simulink model "myAdcDither"  (Simulink 7.3)
settings: Solver=FixedStepDiscrete  StartTime=0.0  StopTime=.1  RelTol=1e-3
values from neighbouring files (symbols this model uses):
  Ts = 1/(handles.clkFreq*1e6)*1e9    [myTimingAnalysis.m]
undefined symbols (not defined in the file or in its folder): overSamp
libraries: dspstat3 x3, commfilt2 x1, dspswit3 x1
settings Model: Creator=acarroll  LastModifiedBy=acarroll
settings DataIOCC: LimitDataPoints=off

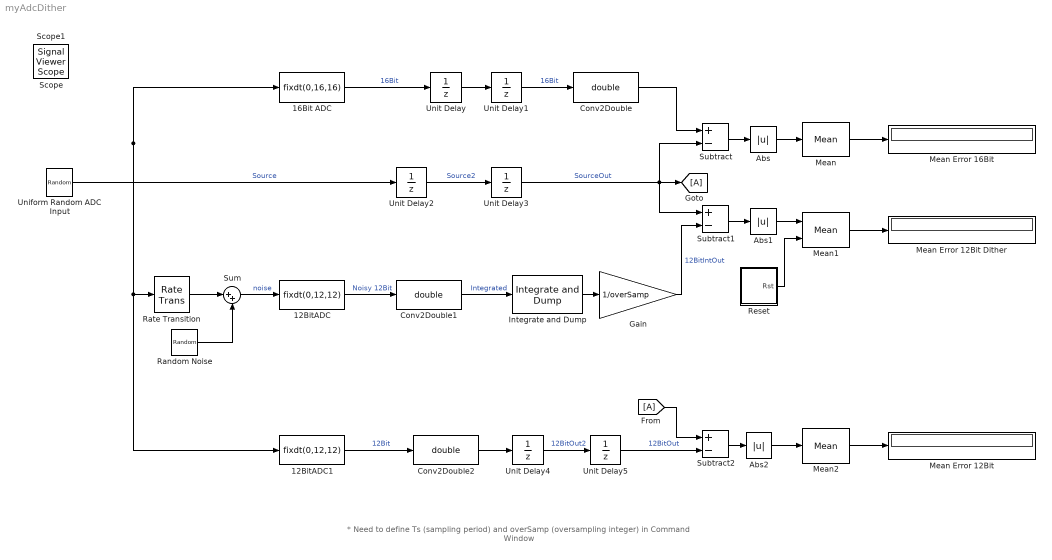
== system myAdcDither ==
  note: * Need to define Ts (sampling period) and overSamp (oversampling integer) in Command Window
  12BitADC : DataTypeConversion  OutDataTypeMode=Specify via dialog  OutDataType=fixdt(0,12,12)  OutDataTypeStr=fixdt(0,12,12)  RndMeth=Nearest  SampleTime=Ts/overSamp  SaturateOnIntegerOverflow=on
  12BitADC1 : DataTypeConversion  OutDataTypeMode=Specify via dialog  OutDataType=fixdt(0,12,12)  OutDataTypeStr=fixdt(0,12,12)  RndMeth=Nearest  SampleTime=Ts  SaturateOnIntegerOverflow=on
  16Bit ADC : DataTypeConversion  OutDataTypeMode=Specify via dialog  OutDataType=fixdt(0,16,16)  OutDataTypeStr=fixdt(0,16,16)  RndMeth=Nearest  SampleTime=Ts  SaturateOnIntegerOverflow=on
  Abs : Abs  OutDataType=fixdt(1, 16)  OutScaling=2^0
  Abs1 : Abs  OutDataType=fixdt(1, 16)  OutScaling=2^0
  Abs2 : Abs  OutDataType=fixdt(1, 16)  OutScaling=2^0
  Conv2Double : DataTypeConversion  OutDataTypeMode=double  OutDataType=fixdt(0,16,16)  OutDataTypeStr=double  SampleTime=Ts
  Conv2Double1 : DataTypeConversion  OutDataTypeMode=double  OutDataType=fixdt(0,16,16)  OutDataTypeStr=double
  Conv2Double2 : DataTypeConversion  OutDataTypeMode=double  OutDataType=fixdt(0,16,16)  OutDataTypeStr=double  SampleTime=Ts
  Gain : Gain  Gain=1/overSamp  ParameterDataType=fixdt(1, 16)  ParameterScaling=2^0  OutDataType=fixdt(1, 16)  OutScaling=2^0
  Integrate and Dump : commfilt2/Integrate and Dump  DialogController=commDDGCreate  DialogControllerArgs=DataTag0  obssamples=overSamp  offsetsamples=0  nodump=off  roundingMode=Convergent  overflowMode=on  outputMode=Binary point scaling  outputWordLength=64  outputFracLength=32
  Mean : dspstat3/Mean  DialogController=dspDDGCreate  DialogControllerArgs=DataTag1  run=on  reset_popup=None  directionMode=Each column  dimension=1  treatSBRowAsCol=on  roiEnable=off  roiType=Rectangles  roiPortion=Entire ROI  roiOutput=Individual statistics for each ROI  roiFlag=off  roundingMode=Floor  overflowMode=off
  Mean Error 12Bit : Display
  Mean Error 12Bit Dither : Display
  Mean Error 16Bit : Display
  Mean1 : dspstat3/Mean  DialogController=dspDDGCreate  DialogControllerArgs=DataTag2  run=on  reset_popup=Rising edge  directionMode=Each column  dimension=1  treatSBRowAsCol=on  roiEnable=off  roiType=Rectangles  roiPortion=Entire ROI  roiOutput=Individual statistics for each ROI  roiFlag=off  roundingMode=Floor  overflowMode=off
  Mean2 : dspstat3/Mean  DialogController=dspDDGCreate  DialogControllerArgs=DataTag3  run=on  reset_popup=None  directionMode=Each column  dimension=1  treatSBRowAsCol=on  roiEnable=off  roiType=Rectangles  roiPortion=Entire ROI  roiOutput=Individual statistics for each ROI  roiFlag=off  roundingMode=Floor  overflowMode=off
  Random Noise : RandomNumber  Variance=(.0002442/2)^2  Seed=5  SampleTime=Ts/overSamp
  Rate Transition : RateTransition
  Reset : Subsystem
  Subtract : Sum  Inputs=+-  OutDataType=fixdt(1, 16)  OutScaling=2^-10
  Subtract1 : Sum  Inputs=+-  OutDataType=fixdt(1, 16)  OutScaling=2^-10
  Subtract2 : Sum  Inputs=+-  OutDataType=fixdt(1, 16)  OutScaling=2^-10
  Sum : Sum  Inputs=|++  OutDataType=fixdt(1, 16)  OutScaling=2^0
  Uniform Random ADC Input : UniformRandomNumber  Minimum=.1  Seed=5  SampleTime=Ts
  Unit Delay{,1..5} (6 alike) : UnitDelay  SampleTime=-1
  Scope : SignalViewerScope  IOType=viewer  ZoomMode=yonly  LegendLocations="602.2778      422.8889      132.6667      62.05556"  RefreshTime=0.035000
      settings: ShowLegends=on
  Scope1 : SignalViewerScope  IOType=viewer  ZoomMode=xonly  LegendLocations="824.2778      504.8889      136.6667      62.05556"  RefreshTime=0.035000
      settings: ShowLegends=on
  wires:
  Uniform Random ADC Input/1 -> 16Bit ADC/1, Unit Delay2/1, Rate Transition/1, 12BitADC1/1  "Source"
  16Bit ADC/1 -> Unit Delay/1  "16Bit"
  Sum/1 -> 12BitADC/1  "noise"
  Random Noise/1 -> Sum/2
  Rate Transition/1 -> Sum/1
  Unit Delay/1 -> Unit Delay1/1
  Unit Delay1/1 -> Conv2Double/1  "16Bit"
  Conv2Double/1 -> Subtract/1
  Unit Delay2/1 -> Unit Delay3/1  "Source2"
  Unit Delay3/1 -> Subtract1/1, Subtract/2, [A]  "SourceOut"
  Subtract/1 -> Abs/1
  Mean/1 -> Mean Error 16Bit/1
  Abs/1 -> Mean/1
  Subtract1/1 -> Abs1/1
  Mean1/1 -> Mean Error 12Bit Dither/1
  Abs1/1 -> Mean1/1
  Gain/1 -> Subtract1/2  "12BitIntOut"
  12BitADC1/1 -> Conv2Double2/1  "12Bit"
  Conv2Double2/1 -> Unit Delay4/1
  Reset/1(Rst) -> Mean1/2
  Unit Delay4/1 -> Unit Delay5/1  "12BitOut2"
  Subtract2/1 -> Abs2/1
  Abs2/1 -> Mean2/1
  Unit Delay5/1 -> Subtract2/2  "12BitOut"
  Mean2/1 -> Mean Error 12Bit/1
  [A] -> Subtract2/1
  Conv2Double1/1 -> Integrate and Dump/1  "Integrated"
  12BitADC/1 -> Conv2Double1/1  "Noisy 12Bit"
  Integrate and Dump/1 -> Gain/1

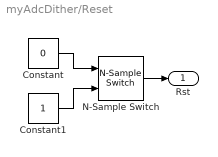
== system myAdcDither/Reset ==
  Constant : Constant  Value=0  OutDataType=fixdt(1, 16)  OutScaling=2^0
  Constant1 : Constant  OutDataType=fixdt(1, 16)  OutScaling=2^0
  N-Sample Switch : dspswit3/N-Sample Switch  SystemSampleTime=-1  N=overSamp  reset=off  TriggerType=Rising edge  Ts=Ts
  Rst : Outport
  wires:
  Constant/1 -> N-Sample Switch/1
  Constant1/1 -> N-Sample Switch/2
  N-Sample Switch/1 -> Rst/1
